simulink model "gm_flatpoint"  (R2022a)
settings: Solver=VariableStepAuto  StartTime=0.0  StopTime=100.0  RelTol=1e-3
settings Model: Creator=Natriya  LastModifiedBy=Natriya
settings OptimizationCC: BlockReduction=off  ConditionallyExecuteInputs=off
settings DebuggingCC: InheritedTsInSrcMsg=none

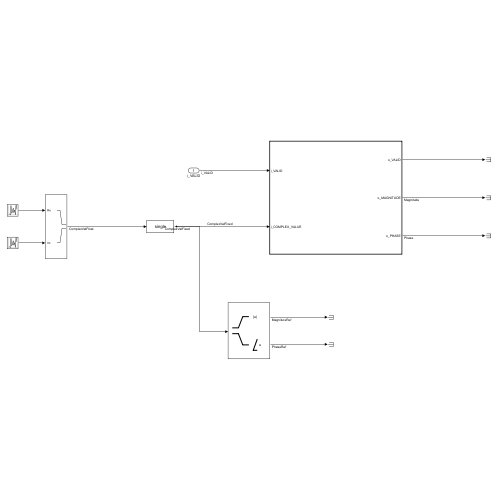
[thumbnail: Simulink's stored preview of the top-level diagram]
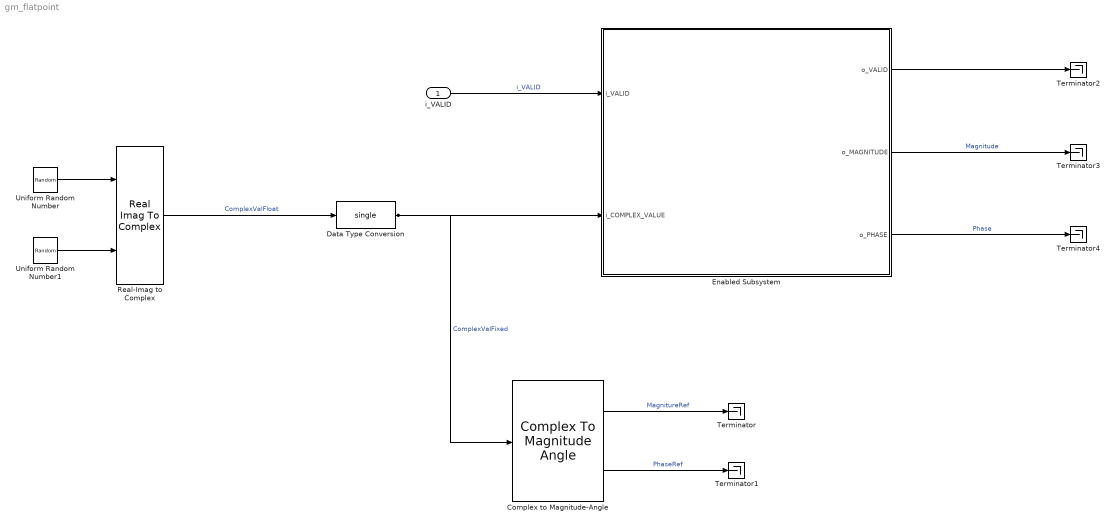
== system gm_flatpoint ==
  i_VALID : Inport
  Complex to Magnitude-Angle : ComplexToMagnitudeAngle
  Data Type Conversion : DataTypeConversion  OutDataTypeStr=single  RndMeth=Round  SaturateOnIntegerOverflow=off
  Enabled Subsystem : Subsystem  TreatAsAtomicUnit=on
  Real-Imag to Complex : RealImagToComplex
  Terminator{,1..4} (5 alike) : Terminator
  Uniform Random Number : UniformRandomNumber  Minimum=-2^(23-1)  Maximum=2^(23-1)-1/2^9  Seed=23  SampleTime=1
  Uniform Random Number1 : UniformRandomNumber  Minimum=-2^(23-1)  Maximum=2^(23-1)-1/2^9  Seed=24  SampleTime=1
  wires:
  Uniform Random Number/1 -> Real-Imag to Complex/1
  i_VALID/1 -> Enabled Subsystem/1(i_VALID)  "i_VALID"
  Uniform Random Number1/1 -> Real-Imag to Complex/2
  Real-Imag to Complex/1 -> Data Type Conversion/1  "ComplexValFloat"
  Enabled Subsystem/3(o_PHASE) -> Terminator4/1  "Phase"
  Complex to Magnitude-Angle/1 -> Terminator/1  "MagnitureRef"
  Enabled Subsystem/1(o_VALID) -> Terminator2/1
  Complex to Magnitude-Angle/2 -> Terminator1/1  "PhaseRef"
  Data Type Conversion/1 -> Enabled Subsystem/2(i_COMPLEX_VALUE), Complex to Magnitude-Angle/1  "ComplexValFixed"
  Enabled Subsystem/2(o_MAGNITUDE) -> Terminator3/1  "Magnitude"

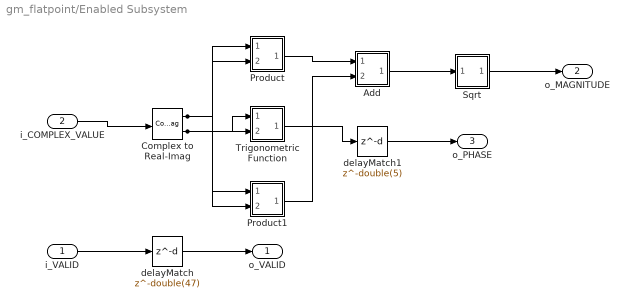
== system gm_flatpoint/Enabled Subsystem ==
  i_VALID : Inport  OutDataTypeStr=double  PortDimensions=1  SampleTime=1
  i_COMPLEX_VALUE : Inport  Port=2  OutDataTypeStr=single  PortDimensions=1  SampleTime=1
      settings: SignalType=complex
  Add : Subsystem
      mask Display: disp('NFP\nadd');
  Complex to Real-Imag : ComplexToRealImag  SampleTime=1
  Product : Subsystem
      mask Display: disp('NFP\nmul');
  Product1 : Subsystem
      mask Display: disp('NFP\nmul');
  Sqrt : Subsystem
      mask Display: disp('NFP\nsqrt');
  Trigonometric Function : Subsystem
      mask Display: disp('NFP\ntrig3');
  delayMatch : Delay  DelayLength=double(47)  InitialCondition=0  SampleTime=1
  delayMatch1 : Delay  DelayLength=double(5)  InitialCondition=0  SampleTime=1
  o_VALID : Outport  SampleTime=1
  o_MAGNITUDE : Outport  Port=2  SampleTime=1  VectorParamsAs1DForOutWhenUnconnected=off
  o_PHASE : Outport  Port=3  SampleTime=1  VectorParamsAs1DForOutWhenUnconnected=off
  wires:
  delayMatch/1 -> o_VALID/1
  i_COMPLEX_VALUE/1 -> Complex to Real-Imag/1
  Complex to Real-Imag/1 -> Trigonometric Function/2(In2), Product/2(In2), Product/1(In1)
  Complex to Real-Imag/2 -> Trigonometric Function/1(In1), Product1/2(In2), Product1/1(In1)
  delayMatch1/1 -> o_PHASE/1
  Add/1(Out1) -> Sqrt/1(In1)
  Product/1(Out1) -> Add/1(In1)
  Product1/1(Out1) -> Add/2(In2)
  Sqrt/1(Out1) -> o_MAGNITUDE/1
  Trigonometric Function/1(Out1) -> delayMatch1/1
  i_VALID/1 -> delayMatch/1

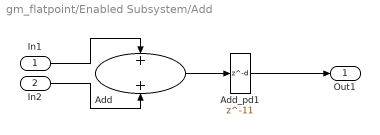
== system gm_flatpoint/Enabled Subsystem/Add ==
  In1 : Inport
  In2 : Inport  Port=2
  Add : Sum  OutDataTypeStr=single  SampleTime=1
  Add_pd1 : Delay  DelayLength=11
  Out1 : Outport
  wires:
  In1/1 -> Add/1
  In2/1 -> Add/2
  Add/1 -> Add_pd1/1
  Add_pd1/1 -> Out1/1

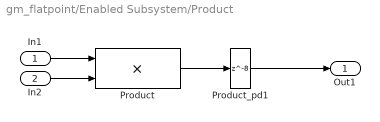
== system gm_flatpoint/Enabled Subsystem/Product ==
  In1 : Inport
  In2 : Inport  Port=2
  Product : Product  Inputs=**  OutDataTypeStr=single  SampleTime=1
  Product_pd1 : Delay  DelayLength=8
  Out1 : Outport
  wires:
  In1/1 -> Product/1
  In2/1 -> Product/2
  Product/1 -> Product_pd1/1
  Product_pd1/1 -> Out1/1

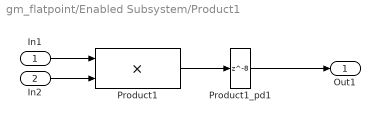
== system gm_flatpoint/Enabled Subsystem/Product1 ==
  In1 : Inport
  In2 : Inport  Port=2
  Product1 : Product  Inputs=**  OutDataTypeStr=single  SampleTime=1
  Product1_pd1 : Delay  DelayLength=8
  Out1 : Outport
  wires:
  In1/1 -> Product1/1
  In2/1 -> Product1/2
  Product1/1 -> Product1_pd1/1
  Product1_pd1/1 -> Out1/1

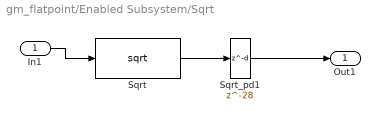
== system gm_flatpoint/Enabled Subsystem/Sqrt ==
  In1 : Inport
  Sqrt : Sqrt  SampleTime=1
  Sqrt_pd1 : Delay  DelayLength=28
  Out1 : Outport
  wires:
  In1/1 -> Sqrt/1
  Sqrt/1 -> Sqrt_pd1/1
  Sqrt_pd1/1 -> Out1/1

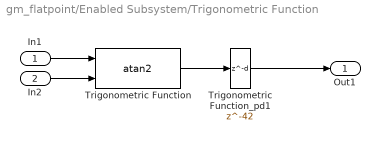
== system gm_flatpoint/Enabled Subsystem/Trigonometric Function ==
  In1 : Inport
  In2 : Inport  Port=2
  Trigonometric Function : Trigonometry  Operator=atan2  SampleTime=1
  Trigonometric Function_pd1 : Delay  DelayLength=42
  Out1 : Outport
  wires:
  In1/1 -> Trigonometric Function/1
  In2/1 -> Trigonometric Function/2
  Trigonometric Function/1 -> Trigonometric Function_pd1/1
  Trigonometric Function_pd1/1 -> Out1/1
